simulink model "sampleModel1622"  (R2023a)
settings: Solver=VariableStepAuto  StartTime=0.0  StopTime=10.0  RelTol=1e-3
libraries: hdlsllib x6, simulink x2
settings Model: Creator=user1  LastModifiedBy=user1

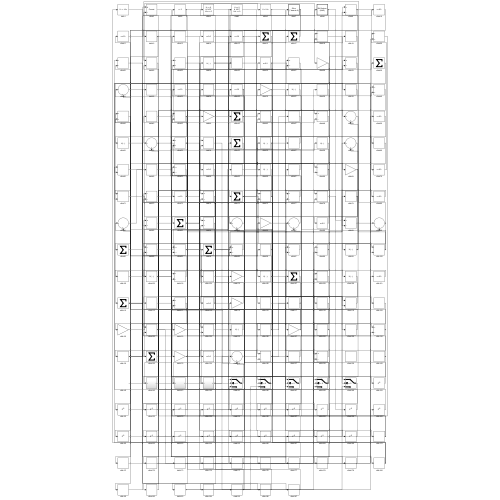
[thumbnail: Simulink's stored preview of the top-level diagram]
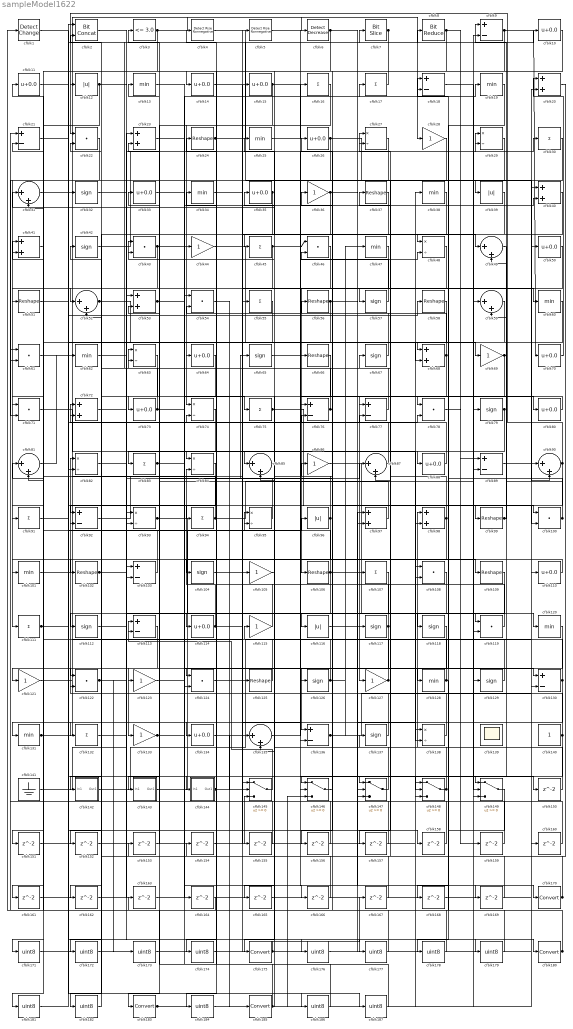
== system sampleModel1622 ==
  cfblk1 : simulink/Logic and Bit Operations/Detect Change  vinit=0  OutDataTypeStr=boolean
      settings: LibrarySourceBlock=|
      | hdlsllib/Logic and Bit
      | Operations/Detect
      | Change
  cfblk{10..11,14..15,26,33,35,50,64,70,73,80,88,110,114,134} (16 alike) : Bias  Bias=0.0  SaturateOnIntegerOverflow=off
  cfblk{22,43,46,54,61,71,78,100,108,119,122,124} (12 alike) : DotProduct  OutDataTypeStr=Inherit: Inherit via internal rule
  cfblk{13,19,25,34,38,47,60,62,101,120,128,131} (12 alike) : MinMax
  cfblk{24,37,51,56,58,66,99,102,106,109,125} (11 alike) : Reshape
  cfblk{9,18,21,76..77,89,92,103,113,130,136} (11 alike) : Sum  Inputs=+-
  cfblk{32,42,57,65,67,79,104,112,117..118,126,129,137} (13 alike) : Signum
  cfblk{28,36,44,69,86,105,115,121,123,127,133} (11 alike) : Gain
  cfblk{16..17,30,45,55,75,83,91,94,107,111,132} (12 alike) : Sum  Inputs=+
  cfblk{12,39,96,116} (4 alike) : Abs  SaturateOnIntegerOverflow=off
  cfblk{31,49,52,59,81,85,87,90,135} (9 alike) : Sum  Inputs=|++
  cfblk{27,29,48,63,74,82,84,93,95,138} (10 alike) : Product  Inputs=*/  RndMeth=Zero  SaturateOnIntegerOverflow=on
  cfblk139 : Scope
      settings: Floating=on
  cfblk140 : Constant  SampleTime=-1
  cfblk141 : Ground
  cfblk142 : Subsystem
      settings: LibrarySourceBlock=|
      | hdlsllib/Ports &
      | Subsystems/Subsystem
  cfblk143 : Subsystem
      settings: LibrarySourceBlock=|
      | hdlsllib/Ports &
      | Subsystems/Subsystem
  cfblk144 : Subsystem
      settings: LibrarySourceBlock=|
      | hdlsllib/Ports &
      | Subsystems/Subsystem
  cfblk{145..149} (5 alike) : Switch  SaturateOnIntegerOverflow=off  InputSameDT=off
  cfblk{150..169} (20 alike) : Delay  SampleTime=1
  cfblk{170,175,180,183,185} (5 alike) : DataTypeConversion  SaturateOnIntegerOverflow=off  RndMeth=Floor
  cfblk{171..174,176..179,181..182,184,186..187} (13 alike) : DataTypeConversion  OutDataTypeStr=uint8  SaturateOnIntegerOverflow=off  RndMeth=Floor
  cfblk2 : hdlsllib/Logic and Bit Operations/Bit Concat  numInputs=2
  cfblk{20,23,40..41,53,68,72,97..98} (9 alike) : Sum
  cfblk3 : hdlsllib/Logic and Bit Operations/Compare To Constant  relop=<=  const=3.0  OutDataTypeStr=boolean
  cfblk4 : hdlsllib/Logic and Bit Operations/Detect Rise Nonnegative  vinit=0  OutDataTypeStr=boolean
  cfblk5 : hdlsllib/Logic and Bit Operations/Detect Rise Nonnegative  vinit=0  OutDataTypeStr=boolean
  cfblk6 : simulink/Logic and Bit Operations/Detect Decrease  vinit=0.0  OutDataTypeStr=boolean
      settings: LibrarySourceBlock=|
      | hdlsllib/Logic and Bit
      | Operations/Detect
      | Decrease
  cfblk7 : hdlsllib/Logic and Bit Operations/Bit Slice  lidx=7  ridx=0
  cfblk8 : hdlsllib/Logic and Bit Operations/Bit Reduce  mode=AND
  wires:
  cfblk78/1 -> cfblk89/1
  cfblk59/1 -> cfblk85/1
  cfblk73/1 -> cfblk7/1, cfblk75/1
  cfblk68/1 -> cfblk127/1, cfblk135/2, cfblk24/1
  cfblk49/1 -> cfblk149/1
  cfblk16/1 -> cfblk74/1
  cfblk131/1 -> cfblk28/1, cfblk95/1, cfblk77/2
  cfblk52/1 -> cfblk68/1, cfblk102/1
  cfblk24/1 -> cfblk8/1, cfblk60/1
  cfblk125/1 -> cfblk115/1
  cfblk90/1 -> cfblk22/1, cfblk146/1
  cfblk148/1 -> cfblk98/1, cfblk72/2
  cfblk126/1 -> cfblk3/1, cfblk47/1
  cfblk145/1 -> cfblk113/1
  cfblk19/1 -> cfblk88/1
  cfblk42/1 -> cfblk29/1
  cfblk146/1 -> cfblk65/1
  cfblk18/1 -> cfblk89/2
  cfblk6/1 -> cfblk49/1, cfblk174/1
  cfblk46/1 -> cfblk106/1
  cfblk74/1 -> cfblk83/1
  cfblk62/1 -> cfblk23/1
  cfblk5/1 -> cfblk170/1
  cfblk9/1 -> cfblk70/1, cfblk126/1
  cfblk86/1 -> cfblk120/1
  cfblk47/1 -> cfblk66/1
  cfblk112/1 -> cfblk119/1
  cfblk17/1 -> cfblk12/1
  cfblk122/1 -> cfblk173/1, cfblk176/1
  cfblk81/1 -> cfblk62/1
  cfblk79/1 -> cfblk128/1, cfblk124/2
  cfblk138/1 -> cfblk82/1
  cfblk106/1 -> cfblk112/1, cfblk119/2, cfblk41/2
  cfblk27/1 -> cfblk111/1
  cfblk117/1 -> cfblk56/1, cfblk181/1
  cfblk56/1 -> cfblk138/2, cfblk184/1
  cfblk82/1 -> cfblk103/1
  cfblk105/1 -> cfblk35/1
  cfblk111/1 -> cfblk58/1, cfblk186/1, cfblk187/1
  cfblk65/1 -> cfblk29/2
  cfblk98/1 -> cfblk132/1, cfblk67/1
  cfblk34/1 -> cfblk48/1
  cfblk118/1 -> cfblk133/1
  cfblk143/1(Out1) -> cfblk96/1
  cfblk26/1 -> cfblk82/2, cfblk39/1
  cfblk37/1 -> cfblk97/2
  cfblk127/1 -> cfblk81/1, cfblk86/1
  cfblk121/1 -> cfblk105/1
  cfblk38/1 -> cfblk183/1
  cfblk80/1 -> cfblk78/1
  cfblk107/1 -> cfblk175/1
  cfblk83/1 -> cfblk44/1, cfblk30/1
  cfblk129/1 -> cfblk37/1
  cfblk8/1 -> cfblk45/1, cfblk159/1
  cfblk100/1 -> cfblk18/1, cfblk49/2
  cfblk132/1 -> cfblk87/1
  cfblk99/1 -> cfblk9/1, cfblk59/2
  cfblk11/1 -> cfblk10/1
  cfblk4/1 -> cfblk90/2
  cfblk76/1 -> cfblk33/1, cfblk156/1
  cfblk44/1 -> cfblk68/2
  cfblk60/1 -> cfblk71/1
  cfblk87/1 -> cfblk43/1
  cfblk71/1 -> cfblk138/1
  cfblk35/1 -> cfblk84/1, cfblk122/1
  cfblk95/1 -> cfblk63/1
  cfblk61/1 -> cfblk32/1
  cfblk114/1 -> cfblk84/2, cfblk17/1
  cfblk92/1 -> cfblk55/1
  cfblk70/1 -> cfblk20/1
  cfblk102/1 -> cfblk27/1, cfblk179/1
  cfblk141/1 -> cfblk103/2
  cfblk55/1 -> cfblk114/1
  cfblk53/1 -> cfblk73/1, cfblk166/1
  cfblk110/1 -> cfblk101/1
  cfblk140/1 -> cfblk87/2, cfblk146/2
  cfblk10/1 -> cfblk14/1
  cfblk113/1 -> cfblk121/1
  cfblk54/1 -> cfblk185/1
  cfblk77/1 -> cfblk42/1
  cfblk142/1(Out1) -> cfblk110/1
  cfblk58/1 -> cfblk142/1(In1)
  cfblk31/1 -> cfblk69/1
  cfblk101/1 -> cfblk15/1
  cfblk93/1 -> cfblk129/1, cfblk147/2
  cfblk119/1 -> cfblk34/1
  cfblk33/1 -> cfblk109/1
  cfblk124/1 -> cfblk125/1
  cfblk13/1 -> cfblk130/1
  cfblk103/1 -> cfblk41/1
  cfblk25/1 -> cfblk16/1
  cfblk43/1 -> cfblk19/1, cfblk93/2
  cfblk136/1 -> cfblk40/1, cfblk117/1
  cfblk109/1 -> cfblk134/1
  cfblk45/1 -> cfblk46/1, cfblk104/1
  cfblk39/1 -> cfblk52/1
  cfblk120/1 -> cfblk136/1
  cfblk32/1 -> cfblk147/1
  cfblk97/1 -> cfblk13/1
  cfblk72/1 -> cfblk94/1
  cfblk128/1 -> cfblk81/2, cfblk168/1
  cfblk14/1 -> cfblk116/1
  cfblk28/1 -> cfblk71/2
  cfblk75/1 -> cfblk100/1, cfblk77/1, cfblk165/1
  cfblk85/1 -> cfblk25/1
  cfblk63/1 -> cfblk92/1
  cfblk7/1 -> cfblk76/1, cfblk171/1
  cfblk130/1 -> cfblk131/1, cfblk72/1
  cfblk2/1 -> cfblk180/1
  cfblk36/1 -> cfblk80/1, cfblk123/1
  cfblk135/1 -> cfblk48/2
  cfblk40/1 -> cfblk64/1
  cfblk104/1 -> cfblk136/2
  cfblk30/1 -> cfblk51/1
  cfblk137/1 -> cfblk53/2
  cfblk51/1 -> cfblk100/2
  cfblk12/1 -> cfblk144/1(In1), cfblk31/2
  cfblk88/1 -> cfblk23/2
  cfblk57/1 -> cfblk36/1
  cfblk94/1 -> cfblk59/1, cfblk79/1, cfblk11/1, cfblk147/3
  cfblk115/1 -> cfblk74/2
  cfblk69/1 -> cfblk149/2, cfblk99/1
  cfblk3/1 -> cfblk6/1, cfblk161/1
  cfblk133/1 -> cfblk78/2, cfblk40/2
  cfblk96/1 -> cfblk124/1, cfblk31/1
  cfblk15/1 -> cfblk118/1, cfblk143/1(In1)
  cfblk89/1 -> cfblk20/2
  cfblk29/1 -> cfblk57/1
  cfblk147/1 -> cfblk137/1
  cfblk22/1 -> cfblk61/2
  cfblk67/1 -> cfblk4/1
  cfblk48/1 -> cfblk91/1
  cfblk1/1 -> cfblk148/2
  cfblk144/1(Out1) -> cfblk145/2, cfblk135/1
  cfblk23/1 -> cfblk150/1
  cfblk150/1 -> cfblk43/2
  cfblk41/1 -> cfblk151/1
  cfblk151/1 -> cfblk98/2
  cfblk84/1 -> cfblk152/1
  cfblk152/1 -> cfblk92/2
  cfblk20/1 -> cfblk153/1
  cfblk153/1 -> cfblk113/2
  cfblk154/1 -> cfblk145/3
  cfblk134/1 -> cfblk155/1
  cfblk155/1 -> cfblk145/1
  cfblk156/1 -> cfblk52/2
  cfblk50/1 -> cfblk157/1
  cfblk157/1 -> cfblk61/1
  cfblk91/1 -> cfblk158/1
  cfblk158/1 -> cfblk63/2
  cfblk159/1 -> cfblk148/1
  cfblk160/1 -> cfblk22/2
  cfblk161/1 -> cfblk9/2
  cfblk66/1 -> cfblk162/1
  cfblk162/1 -> cfblk53/1
  cfblk163/1 -> cfblk148/3
  cfblk123/1 -> cfblk164/1
  cfblk164/1 -> cfblk1/1
  cfblk165/1 -> cfblk95/2
  cfblk166/1 -> cfblk122/2
  cfblk167/1 -> cfblk93/1
  cfblk168/1 -> cfblk130/2
  cfblk116/1 -> cfblk169/1
  cfblk169/1 -> cfblk97/1
  cfblk170/1 -> cfblk27/2, cfblk26/1
  cfblk171/1 -> cfblk5/1
  cfblk108/1 -> cfblk172/1
  cfblk172/1 -> cfblk160/1
  cfblk173/1 -> cfblk108/1
  cfblk174/1 -> cfblk108/2
  cfblk175/1 -> cfblk167/1, cfblk90/1
  cfblk176/1 -> cfblk107/1
  cfblk21/1 -> cfblk177/1
  cfblk177/1 -> cfblk46/2
  cfblk149/1 -> cfblk178/1
  cfblk178/1 -> cfblk21/1
  cfblk179/1 -> cfblk21/2
  cfblk180/1 -> cfblk154/1, cfblk76/2, cfblk18/2
  cfblk181/1 -> cfblk2/1
  cfblk64/1 -> cfblk182/1
  cfblk182/1 -> cfblk2/2
  cfblk183/1 -> cfblk149/3, cfblk50/1
  cfblk184/1 -> cfblk38/1
  cfblk185/1 -> cfblk163/1, cfblk146/3, cfblk85/2
  cfblk186/1 -> cfblk54/1
  cfblk187/1 -> cfblk54/2

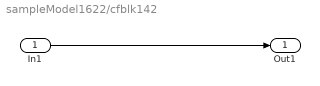
== system sampleModel1622/cfblk142 ==
  In1 : Inport
  Out1 : Outport
  wires:
  In1/1 -> Out1/1

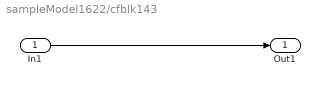
== system sampleModel1622/cfblk143 ==
  In1 : Inport
  Out1 : Outport
  wires:
  In1/1 -> Out1/1

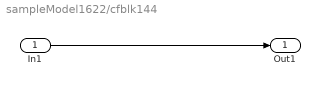
== system sampleModel1622/cfblk144 ==
  In1 : Inport
  Out1 : Outport
  wires:
  In1/1 -> Out1/1
